simulink model ""  (R2019a)
settings: Solver=VariableStepAuto  StartTime=0.0  StopTime=250  RelTol=1e-3
values from neighbouring files (symbols this model uses):
  A = 33    [kalman_dynamic.m]
  a = 0.16    [kalman_dynamic.m]
  Amatd = DSYS.A    [kalman_dynamic.m]
  Bmatd = DSYS.B    [kalman_dynamic.m]
  Cmatd = DSYS.C    [kalman_dynamic.m]
  P0 = 1*eye(2)    [kalman_dynamic.m]
  Ts = 1e-1    (= 0.1)    [kalman_dynamic.m]
  x0 = [h10; h20]    [kalman_dynamic.m]
libraries: R7014E_lib x2, simulink x1
settings Model: Creator=marbla-6  LastModifiedBy=marbla-6
settings SolverCC: ZeroCrossAlgorithm=Adaptive
settings DebuggingCC: IgnoredZcDiagnostic=none

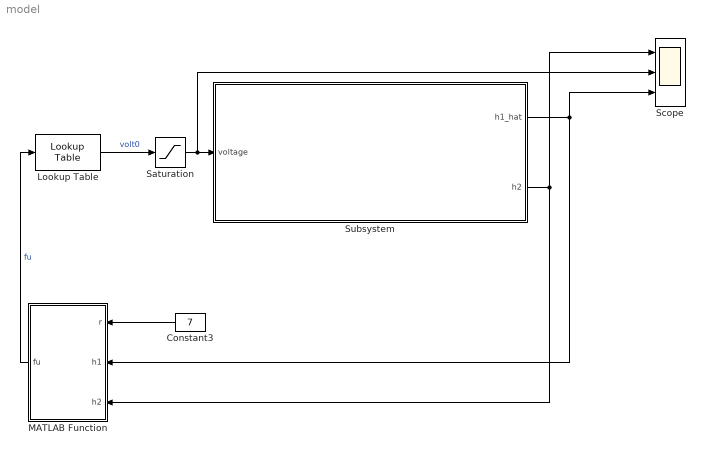
== system model ==
  Constant3 : Constant  Value=7
  Lookup Table : R7014E_lib/Lookup Table  x=[16.47,20.75,24.52,27.63,30.06,32.49,34.8,40.28,48.24,52.43]  y=[0.5,1,1.5,2,2.5,3,3.5,5,8,10]
  MATLAB Function : MATLAB Function  TreatAsAtomicUnit=on
  Saturation : Saturate  UpperLimit=10  LowerLimit=0
  Scope : Scope  NumInputPorts=3
  Subsystem : Subsystem
  wires:
  Constant3/1 -> MATLAB Function/1(r)
  MATLAB Function/1(fu) -> Lookup Table/1  "fu"
  Lookup Table/1 -> Saturation/1  "volt0"
  Subsystem/1(h1_hat) -> Scope/3, MATLAB Function/2(h1)
  Subsystem/2(h2) -> Scope/1, MATLAB Function/3(h2)
  Saturation/1 -> Scope/2, Subsystem/1(voltage)

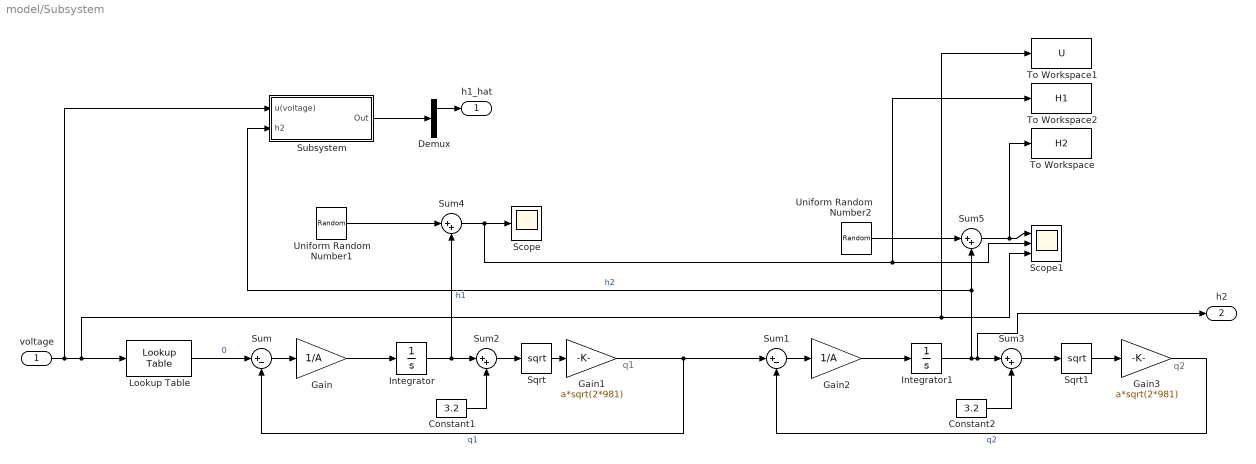
== system model/Subsystem ==
  note: q1
  note: q2
  voltage : Inport
  Constant1 : Constant  Value=3.2
  Constant2 : Constant  Value=3.2
  Demux : Demux  Outputs=2
  Gain : Gain  Gain=1/A
  Gain1 : Gain  Gain=a*sqrt(2*981)
  Gain2 : Gain  Gain=1/A
  Gain3 : Gain  Gain=a*sqrt(2*981)
  Integrator : Integrator  LimitOutput=on  UpperSaturationLimit=15.5  LowerSaturationLimit=0
  Integrator1 : Integrator  LimitOutput=on  UpperSaturationLimit=15.5  LowerSaturationLimit=0
  Lookup Table : R7014E_lib/Lookup Table  x=[0.5,1,1.5,2,2.5,3,3.5,5,8,10]  y=[16.47,20.75,24.52,27.63,30.06,32.49,34.8,40.28,48.24,52.43]
  Scope : Scope
  Scope1 : Scope  NumInputPorts=3
  Sqrt : Sqrt  SaturateOnIntegerOverflow=on
  Sqrt1 : Sqrt  SaturateOnIntegerOverflow=on
  Subsystem : Subsystem
  Sum : Sum  Inputs=|+-
  Sum1 : Sum  Inputs=|+-
  Sum{2..5} (4 alike) : Sum  Inputs=|++
  To Workspace : ToWorkspace  VariableName=H2  SaveFormat=Timeseries  SampleTime=-1
  To Workspace1 : ToWorkspace  VariableName=U  SaveFormat=Timeseries  SampleTime=-1
  To Workspace2 : ToWorkspace  VariableName=H1  SaveFormat=Timeseries  SampleTime=-1
  Uniform Random Number1 : UniformRandomNumber  Minimum=-0.1  Maximum=0.1  SampleTime=0.1
  Uniform Random Number2 : UniformRandomNumber  Minimum=-0.1  Maximum=0.1  SampleTime=0.1
  h1_hat : Outport
  h2 : Outport  Port=2
  wires:
  Lookup Table/1 -> Sum/1  "0"
  Sum3/1 -> Sqrt1/1
  Sum2/1 -> Sqrt/1
  Integrator1/1 -> h2/1, Sum3/1, Subsystem/2(h2), Sum5/2  "h2"
  Gain1/1 -> Sum1/1, Sum/2  "q1"
  Gain2/1 -> Integrator1/1
  Integrator/1 -> Sum2/1, Sum4/2  "h1"
  Constant2/1 -> Sum3/2
  Constant1/1 -> Sum2/2
  voltage/1 -> Subsystem/1(u(voltage)), To Workspace1/1, Scope1/3, Lookup Table/1
  Sum5/1 -> Scope1/1, To Workspace/1
  Sum1/1 -> Gain2/1
  Sqrt1/1 -> Gain3/1
  Gain/1 -> Integrator/1
  Gain3/1 -> Sum1/2  "q2"
  Sqrt/1 -> Gain1/1
  Sum/1 -> Gain/1
  Sum4/1 -> To Workspace2/1, Scope1/2, Scope/1
  Uniform Random Number1/1 -> Sum4/1
  Uniform Random Number2/1 -> Sum5/1
  Subsystem/1(Out) -> Demux/1
  Demux/1 -> h1_hat/1

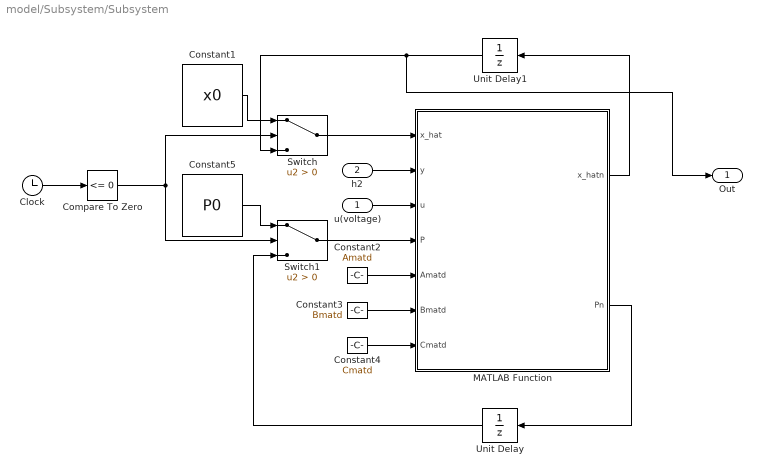
== system model/Subsystem/Subsystem ==
  u(voltage) : Inport
  h2 : Inport  Port=2
  Clock : Clock
  Compare To Zero : simulink/Logic and Bit Operations/Compare To Zero  relop=<=  OutDataTypeStr=boolean
  Constant1 : Constant  Value=x0  VectorParams1D=off  SampleTime=Ts
  Constant2 : Constant  Value=Amatd  VectorParams1D=off  SampleTime=Ts
  Constant3 : Constant  Value=Bmatd  VectorParams1D=off  SampleTime=Ts
  Constant4 : Constant  Value=Cmatd  VectorParams1D=off  SampleTime=Ts
  Constant5 : Constant  Value=P0  VectorParams1D=off  SampleTime=Ts
  MATLAB Function : MATLAB Function  TreatAsAtomicUnit=on
  Switch : Switch  Criteria=u2 > Threshold
  Switch1 : Switch  Criteria=u2 > Threshold
  Unit Delay : UnitDelay  SampleTime=Ts  HasFrameUpgradeWarning=on
  Unit Delay1 : UnitDelay  SampleTime=Ts  HasFrameUpgradeWarning=on
  Out : Outport
  wires:
  h2/1 -> MATLAB Function/2(y)
  u(voltage)/1 -> MATLAB Function/3(u)
  Constant2/1 -> MATLAB Function/5(Amatd)
  Constant4/1 -> MATLAB Function/7(Cmatd)
  Constant3/1 -> MATLAB Function/6(Bmatd)
  MATLAB Function/2(Pn) -> Unit Delay/1
  Constant1/1 -> Switch/1
  Unit Delay1/1 -> Out/1, Switch/3
  Unit Delay/1 -> Switch1/3
  Constant5/1 -> Switch1/1
  Clock/1 -> Compare To Zero/1
  Compare To Zero/1 -> Switch/2, Switch1/2
  Switch1/1 -> MATLAB Function/4(P)
  Switch/1 -> MATLAB Function/1(x_hat)
  MATLAB Function/1(x_hatn) -> Unit Delay1/1

== matlab function Subsystem/Subsystem/MATLAB Function ==
  data: x_hat input; y input; u input; x_hatn output; P input; Pn output; Amatd input; Bmatd input; Cmatd input
function [x_hatn, Pn ] = fcn(x_hat, y, u, P, Amatd, Bmatd, Cmatd)

    Q = 40*eye(2);
    N = 1*eye(2);
    R = 10*eye(2);

    x_hatn = Amatd*x_hat + Bmatd*u;
    Pn = Amatd*P*Amatd' + N*Q*N';  

    K = (Pn*Cmatd')\(Cmatd*Pn*Cmatd' + R);
    y_til = y - Cmatd*x_hatn;
    x_hatn = x_hatn + K*[0; y_til];
    Pn = Pn - K*Cmatd'*Pn;
    
end

== matlab function MATLAB Function ==
  data: r input; h1 input; fu output; h2 input
function fu = fcn(r, h1, h2)

    % h1, h2 are including outlet height
    
    a = 0.16;
    A = 33;
    g = 982;
    h0 = 3.2;
    

    p1=-0.2;
    p2=-0.2;
    

    l_1 = -p1-p2;
    l_2 = p1*p2;
    
    L = [l_2 l_1];
    Lr = l_2;
    
    alpha = -(a^2/A^2)*g*sqrt((h1+h0)/(h2+h0));
    beta = (a/(2*A^2))*sqrt((2*g)/(h1+h0));
    h2_dot = (a/A)*sqrt(2*g)*(sqrt(h1+h0)-sqrt(h2+h0));
    
    x1 = h2;
    x2 = h2_dot;  
    x = [x1; x2];
    
  
    fu = (1/beta)*(-L*x+Lr*r-alpha);
    
end
